simulink model "p7"  (R2020a)
settings: Solver=FixedStepDiscrete  StartTime=0.0  StopTime=25  FixedStep=0.00001  RelTol=1e-3  EnableMultiTasking=on
libraries: commfilt2 x13, commutil2 x9, commrandsrc3 x2
settings Model: Creator=León Mora  LastModifiedBy=León Mora

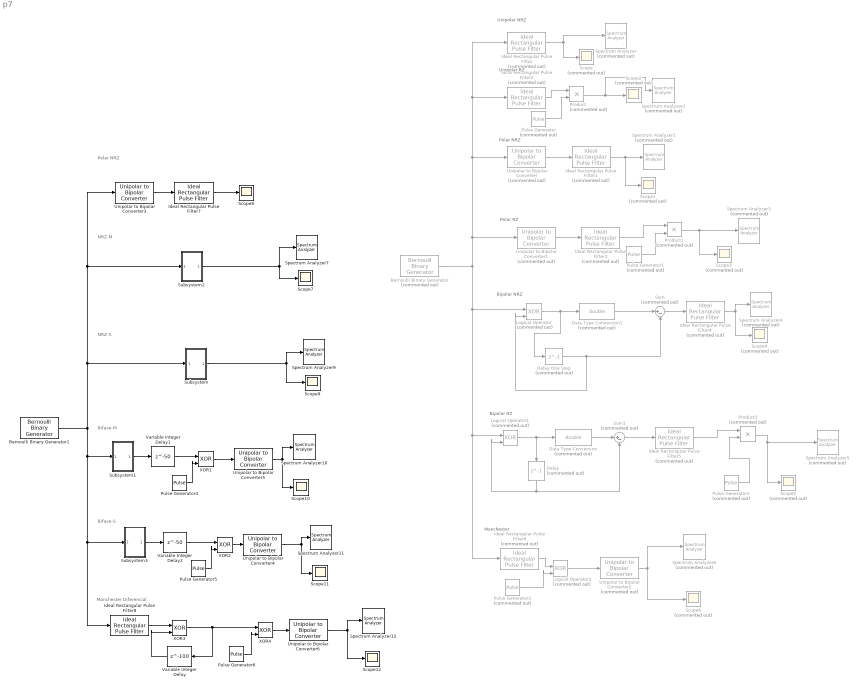
== system p7 ==
  note: Manchester Diferencial
  note: Bifase-S
  note: Bifase-M
  note: NRZ-S
  note: NRZ-M
  note: Manchester
  note: Bipolar RZ
  note: Bipolar NRZ
  note: Polar RZ
  note: Polar NRZ
  note: Unipolar NRZ
  note: Unipolar RZ
  note: Polar NRZ
  Bernoulli Binary Generator : commrandsrc3/Bernoulli Binary Generator  Commented=on  ProbabilityOfZero=0.5  SeedSource=Auto  Seed=0  SampleTime=0.001  SamplesPerFrame=1  OutputDataType=double  SimulateUsing=Interpreted execution
  Bernoulli Binary Generator1 : commrandsrc3/Bernoulli Binary Generator  ProbabilityOfZero=0.5  SeedSource=Auto  Seed=0  SampleTime=0.001  SamplesPerFrame=1  OutputDataType=double  SimulateUsing=Interpreted execution
  Data Type Conversion : DataTypeConversion  Commented=on  OutDataTypeStr=double
  Data Type Conversion1 : DataTypeConversion  Commented=on  OutDataTypeStr=double
  Delay : Delay  Commented=on  DelayLength=1  InitialCondition=0
  Delay One Step : Delay  Commented=on  DelayLength=1
  Ideal Rectangular Pulse Filter{,1..6} (7 alike) : commfilt2/Ideal Rectangular Pulse Filter  Commented=on  pulseLen=100  pulseDelay=0  RateOptions=Allow multirate processing  sampMode=Mute  normCheck=off  normMode=Sum of samples  filterGain=1  saveAsFlag=0  roundingMode=Floor  overflowMode=off  firstCoeffDataTypeStr=Inherit: Same word length as input  firstCoeffMin=[]  firstCoeffMax=[]  firstCoeffLastDataTypeStr=Inherit: Same word length as input  outputDataTypeStr=Inherit: Same as accumulator  outputMin=[]  outputMax=[]  outputLastDataTypeStr=Inherit: Same as accumulator
      settings: SourceProductBaseCode=CM
  Ideal Rectangular Pulse Filter7 : commfilt2/Ideal Rectangular Pulse Filter  pulseLen=100  pulseDelay=0  RateOptions=Allow multirate processing  sampMode=Mute  normCheck=off  normMode=Sum of samples  filterGain=1  saveAsFlag=0  roundingMode=Floor  overflowMode=off  firstCoeffDataTypeStr=Inherit: Same word length as input  firstCoeffMin=[]  firstCoeffMax=[]  firstCoeffLastDataTypeStr=Inherit: Same word length as input  outputDataTypeStr=Inherit: Same as accumulator  outputMin=[]  outputMax=[]  outputLastDataTypeStr=Inherit: Same as accumulator
      settings: SourceProductBaseCode=CM
  Ideal Rectangular Pulse Filter8 : commfilt2/Ideal Rectangular Pulse Filter  pulseLen=100  pulseDelay=0  RateOptions=Allow multirate processing  sampMode=Mute  normCheck=off  normMode=Sum of samples  filterGain=1  saveAsFlag=0  roundingMode=Floor  overflowMode=off  firstCoeffDataTypeStr=Inherit: Same word length as input  firstCoeffMin=[]  firstCoeffMax=[]  firstCoeffLastDataTypeStr=Inherit: Same word length as input  outputDataTypeStr=Inherit: Same as accumulator  outputMin=[]  outputMax=[]  outputLastDataTypeStr=Inherit: Same as accumulator
      settings: SourceProductBaseCode=CM
  Logical Operator : Logic  Commented=on  Operator=XOR  IconShape=distinctive  AllPortsSameDT=off  OutDataTypeStr=boolean
  Logical Operator1 : Logic  Commented=on  Operator=XOR  IconShape=distinctive  AllPortsSameDT=off  OutDataTypeStr=boolean
  Logical Operator2 : Logic  Commented=on  Operator=XOR  IconShape=distinctive  AllPortsSameDT=off  OutDataTypeStr=boolean
  Product : Product  Commented=on
  Product1 : Product  Commented=on
  Product2 : Product  Commented=on
  Pulse Generator{,1..3} (4 alike) : DiscretePulseGenerator  Commented=on  Period=100  PulseWidth=50  SampleTime=0.00001
  Pulse Generator4 : DiscretePulseGenerator  Period=100  PulseWidth=50  SampleTime=0.00001
  Pulse Generator5 : DiscretePulseGenerator  Period=100  PulseWidth=50  SampleTime=0.00001
  Pulse Generator6 : DiscretePulseGenerator  Period=100  PulseWidth=50  SampleTime=0.00001
  Scope{,1..6} (7 alike) : Scope  Commented=on
  Scope{7..12} (6 alike) : Scope
  Spectrum Analyzer{,1..6} (7 alike) : SpectrumAnalyzer  Commented=on
  Spectrum Analyzer{7,9..12} (5 alike) : SpectrumAnalyzer
  Subsystem : Subsystem
      mask Display: disp('NRZ-S')
  Subsystem1 : Subsystem
      mask Display: disp('NRZ-S')
  Subsystem2 : Subsystem
      mask Display: disp('NRZ-M')
  Subsystem3 : Subsystem
      mask Display: disp('NRZ-M')
  Sum : Sum  Commented=on  Inputs=|+-
  Sum1 : Sum  Commented=on  Inputs=|+-
  Unipolar to Bipolar Converter : commutil2/Unipolar to Bipolar Converter  Commented=on  M=2  polarity=Positive  dataType=Inherit via internal rule
  Unipolar to Bipolar Converter1 : commutil2/Unipolar to Bipolar Converter  Commented=on  M=2  polarity=Positive  dataType=Inherit via internal rule
  Unipolar to Bipolar Converter2 : commutil2/Unipolar to Bipolar Converter  Commented=on  M=2  polarity=Positive  dataType=Inherit via internal rule
  Unipolar to Bipolar Converter{3..6} (4 alike) : commutil2/Unipolar to Bipolar Converter  M=2  polarity=Positive  dataType=Inherit via internal rule
  Variable Integer Delay : Delay  DelayLength=100
  Variable Integer Delay1 : Delay  DelayLength=50
  Variable Integer Delay2 : Delay  DelayLength=50
  XOR{1..4} (4 alike) : Logic  Operator=XOR  IconShape=distinctive  AllPortsSameDT=off  OutDataTypeStr=boolean
  wires:
  Ideal Rectangular Pulse Filter/1 -> Scope/1, Spectrum Analyzer/1
  Unipolar to Bipolar Converter/1 -> Ideal Rectangular Pulse Filter1/1
  Ideal Rectangular Pulse Filter1/1 -> Scope1/1, Spectrum Analyzer1/1
  Unipolar to Bipolar Converter1/1 -> Ideal Rectangular Pulse Filter3/1
  Ideal Rectangular Pulse Filter3/1 -> Product1/1
  Pulse Generator1/1 -> Product1/2
  Product1/1 -> Scope3/1, Spectrum Analyzer3/1
  Sum/1 -> Ideal Rectangular Pulse Filter4/1
  Logical Operator/1 -> Delay One Step/1, Data Type Conversion1/1
  Delay One Step/1 -> Logical Operator/2, Sum/2
  Ideal Rectangular Pulse Filter4/1 -> Spectrum Analyzer4/1, Scope4/1
  Logical Operator1/1 -> Delay/1, Data Type Conversion/1
  Sum1/1 -> Ideal Rectangular Pulse Filter5/1
  Ideal Rectangular Pulse Filter5/1 -> Product2/1
  Pulse Generator2/1 -> Product2/2
  Product2/1 -> Spectrum Analyzer5/1, Scope5/1
  Ideal Rectangular Pulse Filter6/1 -> Logical Operator2/1
  Pulse Generator3/1 -> Logical Operator2/2
  Logical Operator2/1 -> Unipolar to Bipolar Converter2/1
  Unipolar to Bipolar Converter2/1 -> Spectrum Analyzer6/1, Scope6/1
  Delay/1 -> Sum1/2, Logical Operator1/2
  Data Type Conversion/1 -> Sum1/1
  Data Type Conversion1/1 -> Sum/1
  Bernoulli Binary Generator/1 -> Logical Operator1/1, Ideal Rectangular Pulse Filter6/1, Logical Operator/1, Ideal Rectangular Pulse Filter2/1, Ideal Rectangular Pulse Filter/1, Unipolar to Bipolar Converter/1, Unipolar to Bipolar Converter1/1
  Ideal Rectangular Pulse Filter2/1 -> Product/1
  Pulse Generator/1 -> Product/2
  Product/1 -> Spectrum Analyzer2/1, Scope2/1
  Ideal Rectangular Pulse Filter7/1 -> Scope8/1
  Unipolar to Bipolar Converter3/1 -> Ideal Rectangular Pulse Filter7/1
  Bernoulli Binary Generator1/1 -> Ideal Rectangular Pulse Filter8/1, Subsystem3/1(In1), Subsystem1/1(In1), Unipolar to Bipolar Converter3/1, Subsystem2/1(In1), Subsystem/1(In1)
  Subsystem/1(Out1) -> Spectrum Analyzer9/1, Scope9/1
  Subsystem1/1(Out1) -> Variable Integer Delay1/1
  Variable Integer Delay1/1 -> XOR1/1
  Pulse Generator4/1 -> XOR1/2
  XOR1/1 -> Unipolar to Bipolar Converter5/1
  Unipolar to Bipolar Converter5/1 -> Scope10/1, Spectrum Analyzer10/1
  Subsystem2/1(Out1) -> Spectrum Analyzer7/1, Scope7/1
  XOR2/1 -> Unipolar to Bipolar Converter4/1
  Pulse Generator5/1 -> XOR2/2
  Unipolar to Bipolar Converter4/1 -> Scope11/1, Spectrum Analyzer11/1
  Variable Integer Delay2/1 -> XOR2/1
  Subsystem3/1(Out1) -> Variable Integer Delay2/1
  Ideal Rectangular Pulse Filter8/1 -> XOR3/1
  Variable Integer Delay/1 -> XOR3/2
  XOR3/1 -> Variable Integer Delay/1, XOR4/1
  Pulse Generator6/1 -> XOR4/2
  XOR4/1 -> Unipolar to Bipolar Converter6/1
  Unipolar to Bipolar Converter6/1 -> Scope12/1, Spectrum Analyzer12/1

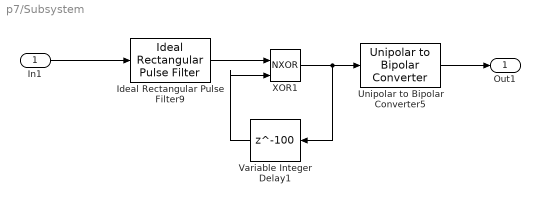
== system p7/Subsystem ==
  In1 : Inport
  Ideal Rectangular Pulse Filter9 : commfilt2/Ideal Rectangular Pulse Filter  pulseLen=100  pulseDelay=0  RateOptions=Allow multirate processing  sampMode=Mute  normCheck=off  normMode=Sum of samples  filterGain=1  saveAsFlag=0  roundingMode=Floor  overflowMode=off  firstCoeffDataTypeStr=Inherit: Same word length as input  firstCoeffMin=[]  firstCoeffMax=[]  firstCoeffLastDataTypeStr=Inherit: Same word length as input  outputDataTypeStr=Inherit: Same as accumulator  outputMin=[]  outputMax=[]  outputLastDataTypeStr=Inherit: Same as accumulator
      settings: SourceProductBaseCode=CM
  Unipolar to Bipolar Converter5 : commutil2/Unipolar to Bipolar Converter  M=2  polarity=Positive  dataType=Inherit via internal rule
  Variable Integer Delay1 : Delay  DelayLength=100
  XOR1 : Logic  Operator=NXOR  IconShape=distinctive  AllPortsSameDT=off  OutDataTypeStr=boolean
  Out1 : Outport
  wires:
  Ideal Rectangular Pulse Filter9/1 -> XOR1/1
  XOR1/1 -> Variable Integer Delay1/1, Unipolar to Bipolar Converter5/1
  Variable Integer Delay1/1 -> XOR1/2
  In1/1 -> Ideal Rectangular Pulse Filter9/1
  Unipolar to Bipolar Converter5/1 -> Out1/1

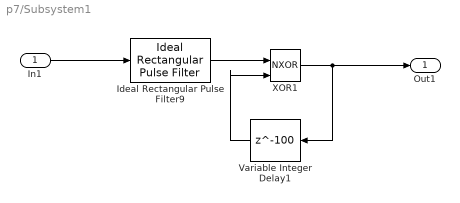
== system p7/Subsystem1 ==
  In1 : Inport
  Ideal Rectangular Pulse Filter9 : commfilt2/Ideal Rectangular Pulse Filter  pulseLen=100  pulseDelay=0  RateOptions=Allow multirate processing  sampMode=Mute  normCheck=off  normMode=Sum of samples  filterGain=1  saveAsFlag=0  roundingMode=Floor  overflowMode=off  firstCoeffDataTypeStr=Inherit: Same word length as input  firstCoeffMin=[]  firstCoeffMax=[]  firstCoeffLastDataTypeStr=Inherit: Same word length as input  outputDataTypeStr=Inherit: Same as accumulator  outputMin=[]  outputMax=[]  outputLastDataTypeStr=Inherit: Same as accumulator
      settings: SourceProductBaseCode=CM
  Variable Integer Delay1 : Delay  DelayLength=100
  XOR1 : Logic  Operator=NXOR  IconShape=distinctive  AllPortsSameDT=off  OutDataTypeStr=boolean
  Out1 : Outport
  wires:
  Ideal Rectangular Pulse Filter9/1 -> XOR1/1
  Variable Integer Delay1/1 -> XOR1/2
  In1/1 -> Ideal Rectangular Pulse Filter9/1
  XOR1/1 -> Out1/1, Variable Integer Delay1/1

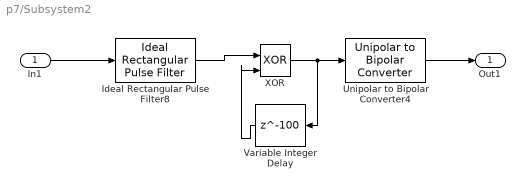
== system p7/Subsystem2 ==
  In1 : Inport
  Ideal Rectangular Pulse Filter8 : commfilt2/Ideal Rectangular Pulse Filter  pulseLen=100  pulseDelay=0  RateOptions=Allow multirate processing  sampMode=Mute  normCheck=off  normMode=Sum of samples  filterGain=1  saveAsFlag=0  roundingMode=Floor  overflowMode=off  firstCoeffDataTypeStr=Inherit: Same word length as input  firstCoeffMin=[]  firstCoeffMax=[]  firstCoeffLastDataTypeStr=Inherit: Same word length as input  outputDataTypeStr=Inherit: Same as accumulator  outputMin=[]  outputMax=[]  outputLastDataTypeStr=Inherit: Same as accumulator
      settings: SourceProductBaseCode=CM
  Unipolar to Bipolar Converter4 : commutil2/Unipolar to Bipolar Converter  M=2  polarity=Positive  dataType=Inherit via internal rule
  Variable Integer Delay : Delay  DelayLength=100
  XOR : Logic  Operator=XOR  IconShape=distinctive  AllPortsSameDT=off  OutDataTypeStr=boolean
  Out1 : Outport
  wires:
  In1/1 -> Ideal Rectangular Pulse Filter8/1
  Ideal Rectangular Pulse Filter8/1 -> XOR/1
  XOR/1 -> Unipolar to Bipolar Converter4/1, Variable Integer Delay/1
  Variable Integer Delay/1 -> XOR/2
  Unipolar to Bipolar Converter4/1 -> Out1/1

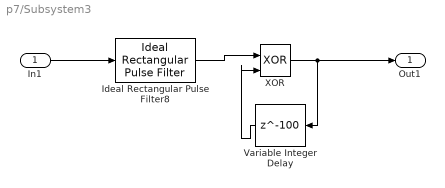
== system p7/Subsystem3 ==
  In1 : Inport
  Ideal Rectangular Pulse Filter8 : commfilt2/Ideal Rectangular Pulse Filter  pulseLen=100  pulseDelay=0  RateOptions=Allow multirate processing  sampMode=Mute  normCheck=off  normMode=Sum of samples  filterGain=1  saveAsFlag=0  roundingMode=Floor  overflowMode=off  firstCoeffDataTypeStr=Inherit: Same word length as input  firstCoeffMin=[]  firstCoeffMax=[]  firstCoeffLastDataTypeStr=Inherit: Same word length as input  outputDataTypeStr=Inherit: Same as accumulator  outputMin=[]  outputMax=[]  outputLastDataTypeStr=Inherit: Same as accumulator
      settings: SourceProductBaseCode=CM
  Variable Integer Delay : Delay  DelayLength=100
  XOR : Logic  Operator=XOR  IconShape=distinctive  AllPortsSameDT=off  OutDataTypeStr=boolean
  Out1 : Outport
  wires:
  In1/1 -> Ideal Rectangular Pulse Filter8/1
  Ideal Rectangular Pulse Filter8/1 -> XOR/1
  Variable Integer Delay/1 -> XOR/2
  XOR/1 -> Out1/1, Variable Integer Delay/1
